simulink model "simullation"  (R2023b)
settings: Solver=VariableStepAuto  StartTime=0.0  StopTime=1000  RelTol=1e-3
model workspace (MAT data in the model file):
  Ip = [0.0088  0  0; 0  0.0088  0; 0  0  0.0044]
  K = [-0.000443603406231  6.73781157753e-21  7.77483629526e-20  -2.2360679775e-05  1.97212558932e-22  4.89230925948e-21; -1.70527086841e-22  -0.000443603406231  5.17001334298e-23  5.35166006497e-24  -2.2360679775e-05  6.43091806088e-23; -1.08514122647e-19  -3.33029792061e-22  -0.000313682946636  -5.39626121661e-21  -4.51886536799e-23  -2.2360679775e-05]
  K_slow = [-4.43592247475e-05  2.07136254246e-21  7.30622127449e-24  -2.2360679775e-07  1.49423035408e-23  -8.57955308484e-26; 3.74861167684e-22  -4.43592247475e-05  2.96582119032e-22  2.07897257759e-24  -2.2360679775e-07  3.98836879416e-24; -1.03139362024e-24  4.10125083945e-24  -3.13667165974e-05  -4.97747355618e-27  1.55658517825e-26  -2.2360679775e-07]
  M = 2
  Nu = [0  0  0; 0  0  0; 0  0  0]
  Nx = [0  0  0; 0  0  0; 0  0  0; 1  0  0; 0  1  0; 0  0  1]
  tracking_angle_required = [0 0.692021234823 1.38404246965 2.07606370447 2.76808493929 3.46010617411 4.15212740894 4.84414864376 5.53616987858 6.2281911134 6.92021234823 7.61223358305 ... (2000 elements, 1000x2)]
libraries: sharedtransform x3, shared6dof x1, aerolibanim x1
settings Model: PacingRate=100  Creator=david  LastModifiedBy=david

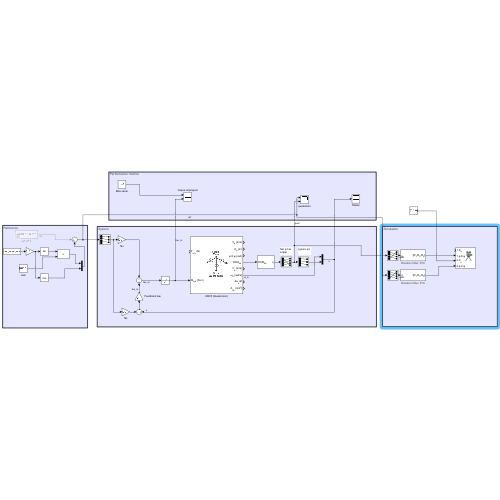
[thumbnail: Simulink's stored preview of the top-level diagram]
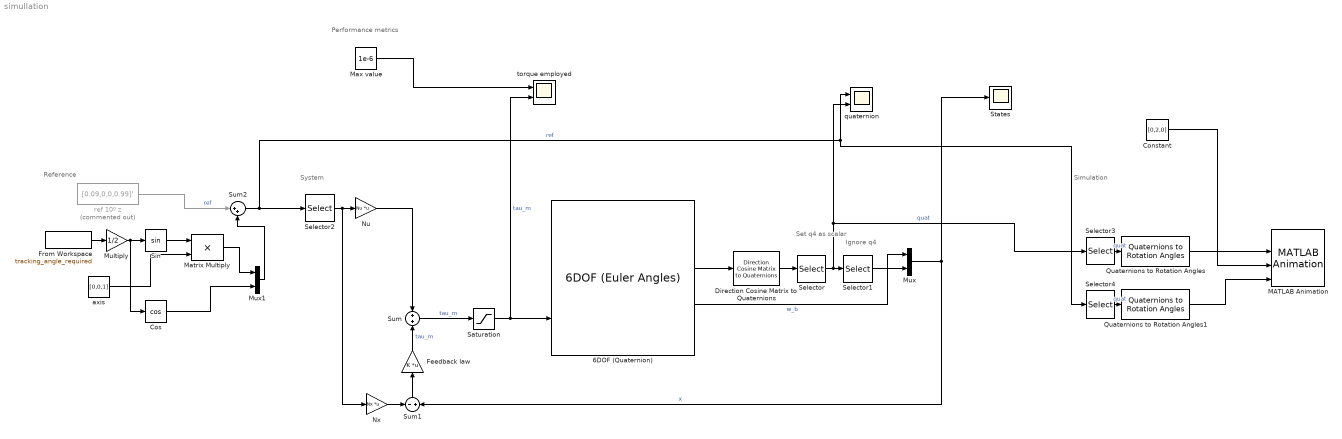
== system simullation ==
  note: Simulation
  note: Performance metrics
  note: Reference
  note: System
  note: Set q4 as scalar
  note: Ignore q4
  6DOF (Quaternion) : shared6dof/6DOF (Euler Angles)  units=Metric (MKS)  mtype=Fixed  rep=Quaternion  xme_0=[0 0 0]  Vm_0=[0 0 0]  eul_0=[0,0,0]  pm_0=[0 0 0]  mass_0=M  mass_e=0.5  mass_f=2.0  inertia=Ip  inertia_e=eye(3)  inertia_f=2*eye(3)  k_quat=1.0  vre_flag=on  abi_flag=off  aMode=0  xme_statename=''  Vm_statename=''  eul_statename=''  quat_statename=''  pm_statename=''  mass_statename=''
      settings: LibrarySourceBlock=aerolib6dof2/6DOF (Quaternion)
  Constant : Constant  Value=[0,2,0]
  Cos : Trigonometry  Operator=cos
  Direction Cosine Matrix to Quaternions : sharedtransform/Direction Cosine Matrix  to Quaternions  aMode=0  action=None  tolerance=eps(2)
      settings: LibrarySourceBlock=|
      | aerolibtransform2/Direction Cosine Matrix
      | to Quaternions
  Feedback law : Gain  Gain=K  Multiplication=Matrix(K*u)
  From Workspace : FromWorkspace  VariableName=tracking_angle_required  SampleTime=-1
  MATLAB Animation : aerolibanim/MATLAB Animation  Tag=Matlab Animation 6 DOF  Vehicles=2  Geometries={'astredwedge.mat','astredwedge.mat'}  BoundingBoxCoordinates=[-50,50,-50,50,-50,50]  CameraOffset=[-150,-50,0]  CameraViewAngle=3  SampleTime=3  FigurePosition=[1,41,1536,7.744000e+02]
  Matrix Multiply : Product
  Max value : Constant  Value=1e-6
  Multiply : Gain  Gain=1/2
  Mux : Mux  Inputs=2
  Mux1 : Mux  Inputs=2
  Nu : Gain  Gain=Nu  Multiplication=Matrix(K*u)
  Nx : Gain  Gain=Nx  Multiplication=Matrix(K*u)
  Quaternions to Rotation Angles : sharedtransform/Quaternions to Rotation Angles  rotationOrder=ZYX  aMode=aMode
  Quaternions to Rotation Angles1 : sharedtransform/Quaternions to Rotation Angles  rotationOrder=ZYX  aMode=aMode
  Saturation : Saturate  UpperLimit=1e-6  LowerLimit=-1e-6
  Selector : Selector  InputPortWidth=4  IndexOptions=Index vector (dialog)  Indices=[2 3 4 1 ]  OutputSizes=1
  Selector1 : Selector  InputPortWidth=4  IndexOptions=Index vector (dialog)  Indices=[1 2 3 ]  OutputSizes=1
  Selector2 : Selector  InputPortWidth=4  IndexOptions=Index vector (dialog)  Indices=[1 2 3 ]  OutputSizes=1
  Selector3 : Selector  InputPortWidth=4  IndexOptions=Index vector (dialog)  Indices=[4 1 2 3 ]  OutputSizes=1
  Selector4 : Selector  InputPortWidth=4  IndexOptions=Index vector (dialog)  Indices=[4 1 2 3 ]  OutputSizes=1
  Sin : Trigonometry
  States : Scope
  Sum : Sum  Inputs=+|+
  Sum1 : Sum  Inputs=-|+
  Sum2 : Sum  Inputs=|++
  axis : Constant  Value=[0,0,1]
  quaternion : Scope  NumInputPorts=2
  ref 10º z : Constant  Commented=on  Value=[0.09,0,0,0.99]'
  torque employed : Scope  NumInputPorts=2
  wires:
  6DOF (Quaternion)/4 -> Direction Cosine Matrix to Quaternions/1
  6DOF (Quaternion)/6 -> Mux/1  "w_b"
  Direction Cosine Matrix to Quaternions/1 -> Selector/1
  Mux/1 -> Sum1/2, States/1  "x"
  Selector/1 -> Selector3/1, quaternion/2, Selector1/1  "quat"
  Selector1/1 -> Mux/2
  Feedback law/1 -> Sum/2  "tau_m"
  Sum/1 -> Saturation/1  "tau_m"
  Max value/1 -> torque employed/1
  Nu/1 -> Sum/1
  Sum1/1 -> Feedback law/1
  Nx/1 -> Sum1/1
  Selector2/1 -> Nx/1, Nu/1
  Quaternions to Rotation Angles1/1 -> MATLAB Animation/4
  Constant/1 -> MATLAB Animation/3
  From Workspace/1 -> Multiply/1
  Sin/1 -> Matrix Multiply/1
  axis/1 -> Matrix Multiply/2
  Multiply/1 -> Cos/1, Sin/1
  Matrix Multiply/1 -> Mux1/1
  Cos/1 -> Mux1/2
  Mux1/1 -> Sum2/2
  ref 10º z/1 -> Sum2/1  "ref"
  Sum2/1 -> Selector4/1, quaternion/1, Selector2/1  "ref"
  Saturation/1 -> torque employed/2, 6DOF (Quaternion)/2  "tau_m"
  Quaternions to Rotation Angles/1 -> MATLAB Animation/2
  Selector3/1 -> Quaternions to Rotation Angles/1  "quat"
  Selector4/1 -> Quaternions to Rotation Angles1/1  "quat"
